simulink model "SystemSimulationPPO"  (R2024b)
settings: Solver=FixedStepAuto  StartTime=0.0  StopTime=TMax  FixedStep=0.01  MaxStep=DT  RelTol=1e-3  EnableMultiTasking=on
undefined symbols (not defined in the file or in its folder): Beta_Array, Cp_Table, Ct_Table, MPC_Implicit, MPC_Lidar, OutList, strmatch, TSR_Array
libraries: simulink_extras x3, rllib x1, matrix_library x1
settings Model: Creator=bjonkman  LastModifiedBy=malth
settings SolverCC: AlgebraicLoopSolver=TrustRegion  AutoInsertRateTranBlk=on
settings DataIOCC: SaveFormat=Array  SignalLoggingSaveFormat=ModelDataLogs  SaveOutput=off  SaveTime=off  ReturnWorkspaceOutputs=off  SignalLoggingName=sigsOut
settings OptimizationCC: ExpressionDepthLimit=2147483647  LifeSpan=inf
settings DebuggingCC: SaveWithParameterizedLinksMsg=none  UnderspecifiedInitializationDetection=Classic  MergeDetectMultiDrivingBlocksExec=none  SignalResolutionControl=TryResolveAllWithWarning  MultiTaskDSMMsg=warning  MultiTaskCondExecSysMsg=none  FcnCallInpInsideContextMsg=warning  UnconnectedInputMsg=warning  UnconnectedOutputMsg=warning  UnconnectedLineMsg=warning  StateNameClashWarn=warning  SFUnexpectedBacktrackingDiag=warning  SFNoUnconditionalDefaultTransitionDiag=warning  SFExecutionAtInitializationDiag=none  UnderSpecifiedDimensionMsg=warning  ArithmeticOperatorsInVariantConditions=warning
settings HardwareCC: ProdBitPerPointer=32  ProdBitPerSizeT=32  ProdBitPerPtrDiffT=32  ProdLargestAtomicFloat=None  ProdIntDivRoundTo=Undefined  ProdEndianess=Unspecified  ProdWordSize=32  ProdHWDeviceType=32-bit Generic  TargetBitPerPointer=64  TargetBitPerSizeT=64  TargetBitPerPtrDiffT=64  TargetLongLongMode=on  TargetIntDivRoundTo=Zero  TargetEndianess=LittleEndian  TargetWordSize=64  TargetHWDeviceType=MATLAB Host  ProdEqTarget=off
settings ModelReferenceCC: EnableRefExpFcnMdlSchedulingChecks=on  PropagateSignalLabelsOutOfModel=off
settings SFSimCC: SimUseLocalCustomCode=off  CustomCodeUndefinedFunction=UseInterfaceOnly
settings RTWCC: RTWUseLocalCustomCode=off  GPUComputeCapability=3.5  DLArmComputeVersion=19.05
settings CodeAppCC: StateflowObjectComments=on
settings GRTTargetCC: TargetLangStandard=C89/C90 (ANSI)  ModelReferenceCompliant=off  ParMdlRefBuildCompliant=off  CompOptLevelCompliant=off  ConcurrentExecutionCompliant=off  CombineOutputUpdateFcns=off  MatFileLogging=off  GRTInterface=on
settings ConfigComp: CovMetricSettings=dw  CovSaveCumulativeToWorkspaceVar=on  CovSaveSingleToWorkspaceVar=on  CovExternalEMLEnable=off

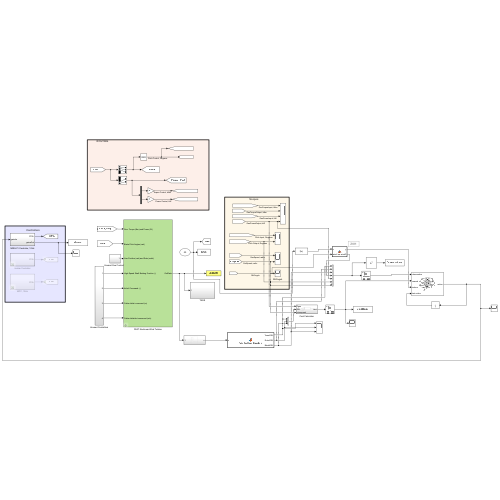
[thumbnail: Simulink's stored preview of the top-level diagram]
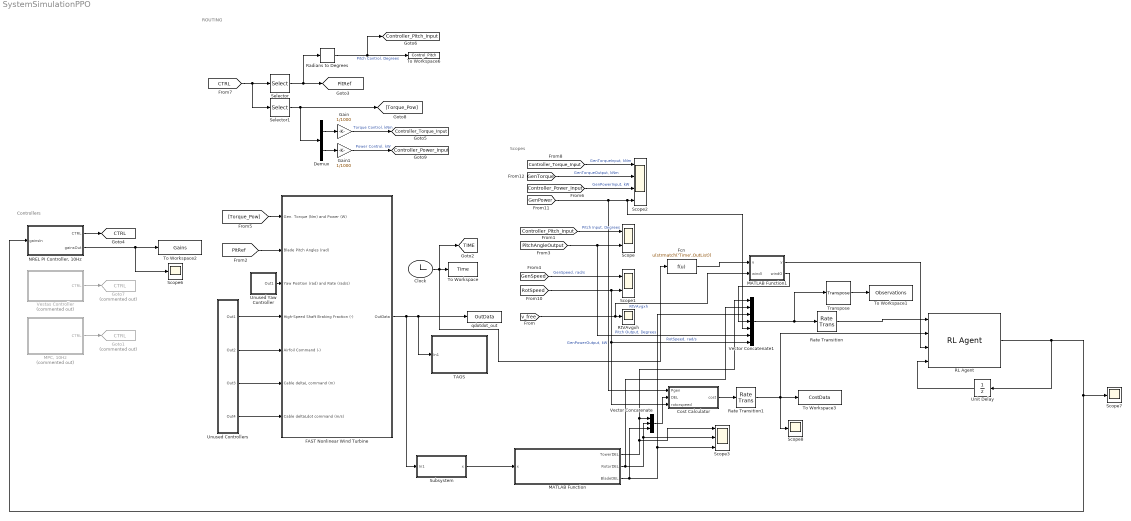
== system SystemSimulationPPO ==
  note: ROUTING
  note: Scopes
  note: Controllers
  Clock : Clock
  Cost Calculator : Subsystem
  Demux : Demux  Outputs=2
  FAST Nonlinear Wind Turbine : Subsystem  mask(FAST Nonlinear Wind Turbine){}
      mask help: This block contains the FAST S-Function.
      mask init:
      | clear FAST_SFunc
  Fcn : Fcn  Expr=u(strmatch('Time',OutList))
  Gain : Gain  Gain=1/1000
  Gain1 : Gain  Gain=1/1000
  Goto1 : Goto  Commented=on  GotoTag=CTRL  TagVisibility=global
  Goto7 : Goto  Commented=on  GotoTag=CTRL  TagVisibility=global
  MATLAB Function : MATLAB Function  TreatAsAtomicUnit=on
  MATLAB Function1 : MATLAB Function  TreatAsAtomicUnit=on
  "MPC, 10Hz" : Subsystem  Commented=on
  "NREL PI Controller, 10Hz" : Subsystem
  RL Agent : rllib/RL Agent  Agent=agent  ExternalActionAsInput=off  ProvideLastAction=on  ProvideCumRwd=off  TreatAsDirectFeedthrough=on  UseStrictObservationDataTypes=off
  Radians to Degrees : simulink_extras/Transformations/Radians to Degrees
  Rate Transition : RateTransition  OutPortSampleTime=0.1
  Rate Transition1 : RateTransition  OutPortSampleTime=0.1
  RtVAvgxh : Scope
  Scope : Scope  NumInputPorts=2
  Scope1 : Scope  NumInputPorts=2
  Scope2 : Scope  NumInputPorts=4
  Scope3 : Scope  NumInputPorts=3
  Scope6 : Scope
  Scope7 : Scope
  Scope8 : Scope
  Selector : Selector  InputPortWidth=5  IndexOptions=Index vector (dialog)  Indices=[1, 2, 3]  OutputSizes=1
  Selector1 : Selector  InputPortWidth=5  IndexOptions=Index vector (dialog)  Indices=[4, 5]  OutputSizes=1
  Subsystem : Subsystem
  TAGS : Subsystem
  To Workspace : ToWorkspace  VariableName=Time  SampleTime=-1
  To Workspace1 : ToWorkspace  VariableName=Observations  SampleTime=-1
      settings: Save2DSignal=2-D array (concatenate along first dimension)
  To Workspace2 : ToWorkspace  VariableName=Gains  SaveFormat=Timeseries  SampleTime=-1
  To Workspace3 : ToWorkspace  VariableName=CostData  SampleTime=-1
  To Workspace6 : ToWorkspace  VariableName=Control_Pitch  SampleTime=-1
  Transpose : matrix_library/Transpose
  Unit Delay : UnitDelay  SampleTime=-1  HasFrameUpgradeWarning=on
  Unused Controllers : Subsystem
  Unused Yaw Controller : Subsystem
  Vector Concatenate : Concatenate  NumInputs=3  Mode=Multidimensional array  ConcatenateDimension=2
  Vector Concatenate1 : Concatenate  NumInputs=7  Mode=Multidimensional array  ConcatenateDimension=2
  Vestas Controller : Subsystem  Commented=on  TreatAsAtomicUnit=on  SystemSampleTime=0.01
  qdotdot_out : ToWorkspace  VariableName=OutData  SampleTime=-1
  tag scope: CTRL=global, Controller_Pitch_Input=global, Controller_Power_Input=global, Controller_Torque_Input=global, PitRef=global, TIME=global
  wires:
  Clock/1 -> [TIME], To Workspace/1, Fcn/1
  Unused Yaw Controller/1(Out1) -> FAST Nonlinear Wind Turbine/3(Yaw Position (rad) and Rate (rad/s))
  [PitRef] -> FAST Nonlinear Wind Turbine/2(Blade Pitch Angles (rad))
  [PitchAngleOutput] -> Vector Concatenate1/6, Scope/2  "Pitch Output, Degrees"
  [GenSpeed] -> Scope1/1  "GenSpeed, rad/s"
  [RotSpeed] -> Cost Calculator/3(rotorspeed), Vector Concatenate1/7, Scope1/2  "RotSpeed, rad/s"
  [v_free] -> RtVAvgxh/1, MATLAB Function1/2(windI)  "RtVAvgxh"
  "NREL PI Controller, 10Hz"/1(CTRL) -> [CTRL]
  [Controller_Pitch_Input] -> Scope/1  "Pitch Input, Degrees"
  Unused Controllers/1(Out1) -> FAST Nonlinear Wind Turbine/4(High-Speed Shaft Braking Fraction (-))
  Unused Controllers/2(Out2) -> FAST Nonlinear Wind Turbine/5(Airfoil Command (-))
  Unused Controllers/3(Out3) -> FAST Nonlinear Wind Turbine/6(Cable deltaL command (m))
  Unused Controllers/4(Out4) -> FAST Nonlinear Wind Turbine/7(Cable deltaLdot command (m/s))
  "MPC, 10Hz"/1(CTRL) -> Goto1/1
  Vestas Controller/1(CTRL) -> Goto7/1
  [Torque_Pow] -> FAST Nonlinear Wind Turbine/1(Gen. Torque (Nm) and Power (W))
  [CTRL] -> Selector1/1, Selector/1
  Selector/1 -> Radians to Degrees/1, [PitRef]
  Radians to Degrees/1 -> [Controller_Pitch_Input], To Workspace6/1  "Pitch Control, Degrees"
  Selector1/1 -> Demux/1, [Torque_Pow]
  [GenTorque] -> Scope2/2  "GenTorqueOutput, kNm"
  [GenPower] -> Cost Calculator/1(Pgen), Vector Concatenate1/5, Scope2/4  "GenPowerOutput, kW"
  Demux/1 -> Gain/1
  [Controller_Power_Input] -> Scope2/3  "GenPowerInput, kW"
  [Controller_Torque_Input] -> Scope2/1  "GenTorqueInput, kNm"
  Gain/1 -> [Controller_Torque_Input]  "Torque Control, kNm"
  Gain1/1 -> [Controller_Power_Input]  "Power Control, kW"
  Demux/2 -> Gain1/1
  Subsystem/1(x) -> MATLAB Function/1(x)
  Vector Concatenate/1 -> Cost Calculator/2(DEL)
  MATLAB Function/1(TowerDEL) -> Scope3/1, Vector Concatenate1/1, Vector Concatenate/1
  MATLAB Function/2(RotorDEL) -> Vector Concatenate1/2, Scope3/2, Vector Concatenate/2
  MATLAB Function/3(BladeDEL) -> Vector Concatenate/3, Scope3/3, Vector Concatenate1/3
  "NREL PI Controller, 10Hz"/2(gainsOut) -> Scope6/1, To Workspace2/1
  RL Agent/1 -> Unit Delay/1, "NREL PI Controller, 10Hz"/1(gainsIn), Scope7/1
  Transpose/1 -> To Workspace1/1
  FAST Nonlinear Wind Turbine/1(OutData) -> qdotdot_out/1, TAGS/1(In1), Subsystem/1(In1)
  Vector Concatenate1/1 -> Rate Transition/1, Transpose/1
  Cost Calculator/1(cost) -> Rate Transition1/1
  Rate Transition/1 -> RL Agent/1
  Rate Transition1/1 -> RL Agent/2, To Workspace3/1, Scope8/1
  MATLAB Function1/1(y) -> RL Agent/3
  Fcn/1 -> MATLAB Function1/1(u)
  MATLAB Function1/2(windO) -> Vector Concatenate1/4
  Unit Delay/1 -> RL Agent/4

== system SystemSimulationPPO/Cost Calculator ==
  Pgen : Inport
  DEL : Inport  Port=2
  rotorspeed : Inport  Port=3
  MATLAB Function : MATLAB Function  TreatAsAtomicUnit=on
  cost : Outport
  wires:
  Pgen/1 -> MATLAB Function/2(Pgen)
  DEL/1 -> MATLAB Function/1(DEL)
  MATLAB Function/1(cost) -> cost/1
  rotorspeed/1 -> MATLAB Function/3(rotorspeed)

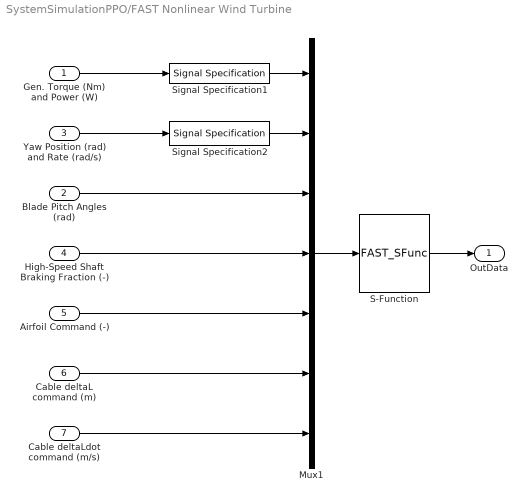
== system SystemSimulationPPO/FAST Nonlinear Wind Turbine ==
  Gen. Torque (Nm) and Power (W) : Inport
  Blade Pitch Angles (rad) : Inport  Port=2
  Yaw Position (rad) and Rate (rad/s) : Inport  Port=3
  High-Speed Shaft Braking Fraction (-) : Inport  Port=4
  Airfoil Command (-) : Inport  Port=5
  Cable deltaL command (m) : Inport  Port=6
  Cable deltaLdot command (m/s) : Inport  Port=7
  Mux1 : Mux  Inputs=7
  S-Function : S-Function  FunctionName=FAST_SFunc  Parameters=FAST_InputFileName, TMax, 0  SFunctionDeploymentMode=off  EnableBusSupport=off
  Signal Specification1 : SignalSpecification  OutDataTypeStr=double  Dimensions=2
  Signal Specification2 : SignalSpecification  OutDataTypeStr=double  Dimensions=2
  OutData : Outport
  wires:
  Gen. Torque (Nm) and Power (W)/1 -> Signal Specification1/1
  S-Function/1 -> OutData/1
  Mux1/1 -> S-Function/1
  Blade Pitch Angles (rad)/1 -> Mux1/3
  Yaw Position (rad) and Rate (rad/s)/1 -> Signal Specification2/1
  Signal Specification1/1 -> Mux1/1
  Signal Specification2/1 -> Mux1/2
  High-Speed Shaft Braking Fraction (-)/1 -> Mux1/4
  Airfoil Command (-)/1 -> Mux1/5
  Cable deltaL command (m)/1 -> Mux1/6
  Cable deltaLdot command (m/s)/1 -> Mux1/7

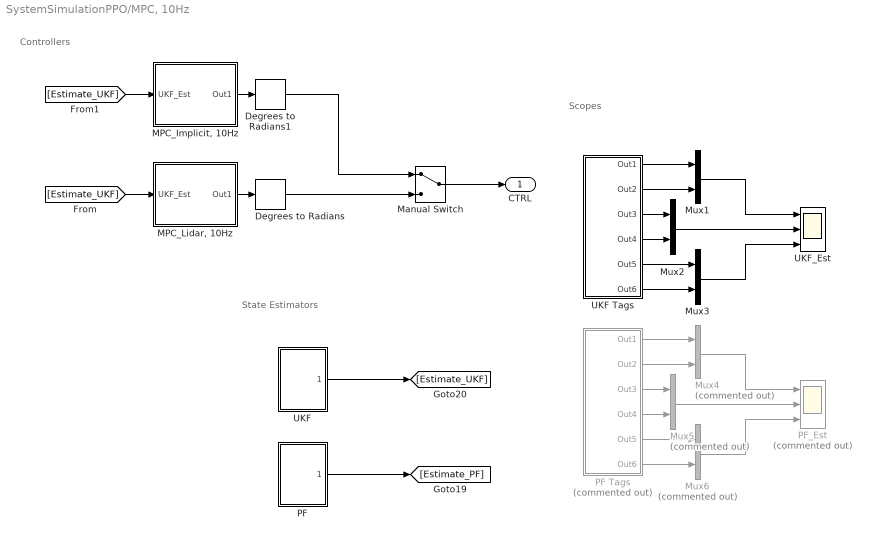
== system SystemSimulationPPO/MPC, 10Hz ==
  note: State Estimators
  note: Scopes
  note: Controllers
  Degrees to Radians : simulink_extras/Transformations/Degrees to Radians
  Degrees to Radians1 : simulink_extras/Transformations/Degrees to Radians
  "MPC_Implicit, 10Hz" : Subsystem
  "MPC_Lidar, 10Hz" : Subsystem
  Manual Switch : ManualSwitch
  Mux1 : Mux  Inputs=2
  Mux2 : Mux  Inputs=2
  Mux3 : Mux  Inputs=2
  Mux4 : Mux  Commented=on  Inputs=2
  Mux5 : Mux  Commented=on  Inputs=2
  Mux6 : Mux  Commented=on  Inputs=2
  PF : Subsystem
  PF Tags : Subsystem  Commented=on
  PF_Est : Scope  Commented=on  NumInputPorts=3
  UKF : Subsystem
  UKF Tags : Subsystem
  UKF_Est : Scope  NumInputPorts=3
  CTRL : Outport
  wires:
  UKF/1(estimate) -> [Estimate_UKF]
  PF/1(estimate) -> [Estimate_PF]
  "MPC_Implicit, 10Hz"/1(Out1) -> Degrees to Radians1/1
  Degrees to Radians1/1 -> Manual Switch/1
  "MPC_Lidar, 10Hz"/1(Out1) -> Degrees to Radians/1
  Degrees to Radians/1 -> Manual Switch/2
  Manual Switch/1 -> CTRL/1
  [Estimate_UKF] -> "MPC_Lidar, 10Hz"/1(UKF_Est)
  [Estimate_UKF] -> "MPC_Implicit, 10Hz"/1(UKF_Est)
  Mux2/1 -> UKF_Est/2
  Mux4/1 -> PF_Est/1
  PF Tags/3(Out3) -> Mux5/1
  Mux6/1 -> PF_Est/3
  PF Tags/1(Out1) -> Mux4/1
  PF Tags/4(Out4) -> Mux5/2
  Mux5/1 -> PF_Est/2
  UKF Tags/2(Out2) -> Mux1/2
  PF Tags/5(Out5) -> Mux6/1
  Mux3/1 -> UKF_Est/3
  UKF Tags/5(Out5) -> Mux3/1
  UKF Tags/4(Out4) -> Mux2/2
  UKF Tags/1(Out1) -> Mux1/1
  Mux1/1 -> UKF_Est/1
  PF Tags/2(Out2) -> Mux4/2
  UKF Tags/3(Out3) -> Mux2/1
  UKF Tags/6(Out6) -> Mux3/2
  PF Tags/6(Out6) -> Mux6/2

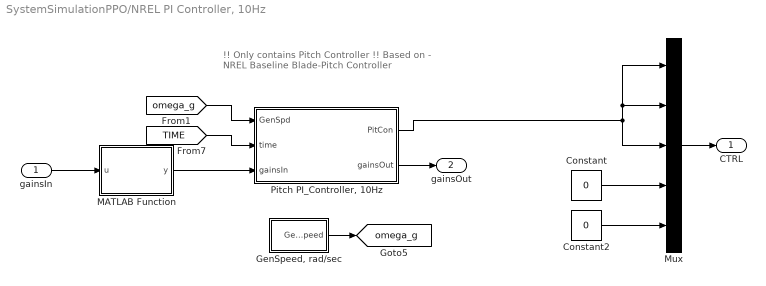
== system SystemSimulationPPO/NREL PI Controller, 10Hz ==
  note: !! Only contains Pitch Controller !!
      |
      | Based on
      | - NREL Baseline Blade-Pitch Controller
  gainsIn : Inport
  Constant : Constant  Value=0
  Constant2 : Constant  Value=0
  "GenSpeed, rad/sec" : Subsystem
  MATLAB Function : MATLAB Function  TreatAsAtomicUnit=on
  Mux : Mux  Inputs=5
  "Pitch PI_Controller, 10Hz" : MATLAB Function  TreatAsAtomicUnit=on
  CTRL : Outport
  gainsOut : Outport  Port=2
  tag scope: omega_g=global
  wires:
  [omega_g] -> "Pitch PI_Controller, 10Hz"/1(GenSpd)
  [TIME] -> "Pitch PI_Controller, 10Hz"/2(time)
  "Pitch PI_Controller, 10Hz"/1(PitCon) -> Mux/3, Mux/2, Mux/1
  Mux/1 -> CTRL/1
  "GenSpeed, rad/sec"/1(GenSpeed) -> [omega_g]
  Constant/1 -> Mux/4
  Constant2/1 -> Mux/5
  gainsIn/1 -> MATLAB Function/1(u)
  "Pitch PI_Controller, 10Hz"/2(gainsOut) -> gainsOut/1
  MATLAB Function/1(y) -> "Pitch PI_Controller, 10Hz"/3(gainsIn)

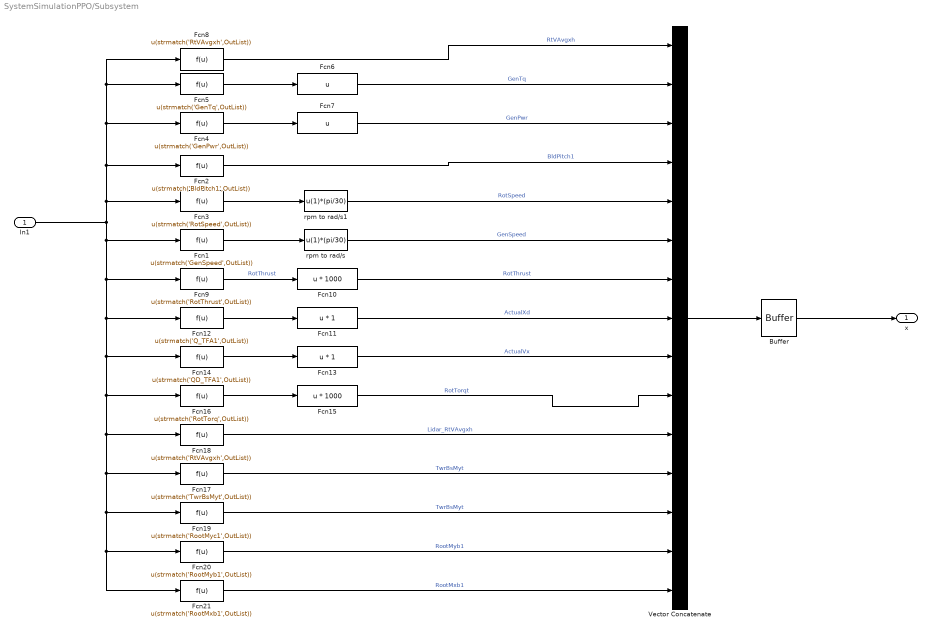
== system SystemSimulationPPO/Subsystem ==
  In1 : Inport
  Buffer : Buffer  N=10  V=9  OutputFrames=off
  Fcn1 : Fcn  Expr=u(strmatch('GenSpeed',OutList))
  Fcn10 : Fcn  Expr=u * 1000
  Fcn11 : Fcn  Expr=u * 1
  Fcn12 : Fcn  Expr=u(strmatch('Q_TFA1',OutList))
  Fcn13 : Fcn  Expr=u * 1
  Fcn14 : Fcn  Expr=u(strmatch('QD_TFA1',OutList))
  Fcn15 : Fcn  Expr=u * 1000
  Fcn16 : Fcn  Expr=u(strmatch('RotTorq',OutList))
  Fcn17 : Fcn  Expr=u(strmatch('TwrBsMyt',OutList))
  Fcn18 : Fcn  Expr=u(strmatch('RtVAvgxh',OutList))
  Fcn19 : Fcn  Expr=u(strmatch('RootMyc1',OutList))
  Fcn2 : Fcn  Expr=u(strmatch('BldPitch1',OutList))
  Fcn20 : Fcn  Expr=u(strmatch('RootMyb1',OutList))
  Fcn21 : Fcn  Expr=u(strmatch('RootMxb1',OutList))
  Fcn3 : Fcn  Expr=u(strmatch('RotSpeed',OutList))
  Fcn4 : Fcn  Expr=u(strmatch('GenPwr',OutList))
  Fcn5 : Fcn  Expr=u(strmatch('GenTq',OutList))
  Fcn6 : Fcn  Expr=u
  Fcn7 : Fcn  Expr=u
  Fcn8 : Fcn  Expr=u(strmatch('RtVAvgxh',OutList))
  Fcn9 : Fcn  Expr=u(strmatch('RotThrust',OutList))
  Vector Concatenate : Concatenate  NumInputs=15  Mode=Multidimensional array  ConcatenateDimension=2
  rpm to rad/s : Fcn  Expr=u(1)*(pi/30)
  rpm to rad/s1 : Fcn  Expr=u(1)*(pi/30)
  x : Outport
  wires:
  Fcn16/1 -> Fcn15/1
  Fcn8/1 -> Vector Concatenate/1  "RtVAvgxh"
  Fcn6/1 -> Vector Concatenate/2  "GenTq"
  Fcn4/1 -> Fcn7/1
  In1/1 -> Fcn8/1, Fcn5/1, Fcn4/1, Fcn2/1, Fcn3/1, Fcn21/1, Fcn20/1, Fcn19/1, Fcn17/1, Fcn18/1, Fcn16/1, Fcn14/1, Fcn12/1, Fcn9/1, Fcn1/1
  Fcn14/1 -> Fcn13/1
  Fcn17/1 -> Vector Concatenate/12  "TwrBsMyt"
  rpm to rad/s/1 -> Vector Concatenate/6  "GenSpeed"
  Fcn5/1 -> Fcn6/1
  Fcn13/1 -> Vector Concatenate/9  "ActualVx"
  Fcn1/1 -> rpm to rad/s/1
  Fcn18/1 -> Vector Concatenate/11  "Lidar_RtVAvgxh"
  Fcn19/1 -> Vector Concatenate/13  "TwrBsMyt"
  Fcn10/1 -> Vector Concatenate/7  "RotThrust"
  rpm to rad/s1/1 -> Vector Concatenate/5  "RotSpeed"
  Fcn20/1 -> Vector Concatenate/14  "RootMyb1"
  Fcn12/1 -> Fcn11/1
  Fcn11/1 -> Vector Concatenate/8  "ActualXd"
  Fcn15/1 -> Vector Concatenate/10  "RotTorqt"
  Fcn9/1 -> Fcn10/1  "RotThrust"
  Fcn7/1 -> Vector Concatenate/3  "GenPwr"
  Fcn2/1 -> Vector Concatenate/4  "BldPitch1"
  Fcn21/1 -> Vector Concatenate/15  "RootMxb1"
  Fcn3/1 -> rpm to rad/s1/1
  Vector Concatenate/1 -> Buffer/1
  Buffer/1 -> x/1

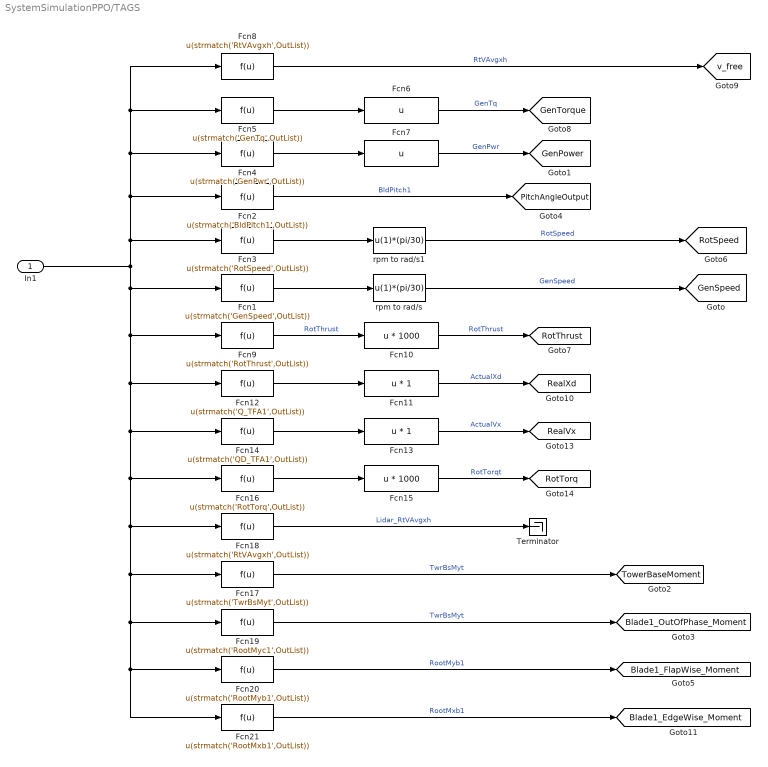
== system SystemSimulationPPO/TAGS ==
  In1 : Inport
  Fcn1 : Fcn  Expr=u(strmatch('GenSpeed',OutList))
  Fcn10 : Fcn  Expr=u * 1000
  Fcn11 : Fcn  Expr=u * 1
  Fcn12 : Fcn  Expr=u(strmatch('Q_TFA1',OutList))
  Fcn13 : Fcn  Expr=u * 1
  Fcn14 : Fcn  Expr=u(strmatch('QD_TFA1',OutList))
  Fcn15 : Fcn  Expr=u * 1000
  Fcn16 : Fcn  Expr=u(strmatch('RotTorq',OutList))
  Fcn17 : Fcn  Expr=u(strmatch('TwrBsMyt',OutList))
  Fcn18 : Fcn  Expr=u(strmatch('RtVAvgxh',OutList))
  Fcn19 : Fcn  Expr=u(strmatch('RootMyc1',OutList))
  Fcn2 : Fcn  Expr=u(strmatch('BldPitch1',OutList))
  Fcn20 : Fcn  Expr=u(strmatch('RootMyb1',OutList))
  Fcn21 : Fcn  Expr=u(strmatch('RootMxb1',OutList))
  Fcn3 : Fcn  Expr=u(strmatch('RotSpeed',OutList))
  Fcn4 : Fcn  Expr=u(strmatch('GenPwr',OutList))
  Fcn5 : Fcn  Expr=u(strmatch('GenTq',OutList))
  Fcn6 : Fcn  Expr=u
  Fcn7 : Fcn  Expr=u
  Fcn8 : Fcn  Expr=u(strmatch('RtVAvgxh',OutList))
  Fcn9 : Fcn  Expr=u(strmatch('RotThrust',OutList))
  Terminator : Terminator
  rpm to rad/s : Fcn  Expr=u(1)*(pi/30)
  rpm to rad/s1 : Fcn  Expr=u(1)*(pi/30)
  tag scope: Blade1_EdgeWise_Moment=global, Blade1_FlapWise_Moment=global, Blade1_OutOfPhase_Moment=global, GenPower=global, GenSpeed=global, GenTorque=global, PitchAngleOutput=global, RealVx=global, RealXd=global, RotSpeed=global, RotThrust=global, RotTorq=global, TowerBaseMoment=global, v_free=global
  wires:
  rpm to rad/s/1 -> [GenSpeed]  "GenSpeed"
  Fcn1/1 -> rpm to rad/s/1
  Fcn3/1 -> rpm to rad/s1/1
  Fcn11/1 -> [RealXd]  "ActualXd"
  In1/1 -> Fcn8/1, Fcn5/1, Fcn4/1, Fcn2/1, Fcn3/1, Fcn21/1, Fcn20/1, Fcn19/1, Fcn17/1, Fcn18/1, Fcn16/1, Fcn14/1, Fcn12/1, Fcn9/1, Fcn1/1
  Fcn7/1 -> [GenPower]  "GenPwr"
  Fcn16/1 -> Fcn15/1
  Fcn10/1 -> [RotThrust]  "RotThrust"
  Fcn6/1 -> [GenTorque]  "GenTq"
  rpm to rad/s1/1 -> [RotSpeed]  "RotSpeed"
  Fcn8/1 -> [v_free]  "RtVAvgxh"
  Fcn5/1 -> Fcn6/1
  Fcn13/1 -> [RealVx]  "ActualVx"
  Fcn4/1 -> Fcn7/1
  Fcn14/1 -> Fcn13/1
  Fcn15/1 -> [RotTorq]  "RotTorqt"
  Fcn2/1 -> [PitchAngleOutput]  "BldPitch1"
  Fcn9/1 -> Fcn10/1  "RotThrust"
  Fcn12/1 -> Fcn11/1
  Fcn18/1 -> Terminator/1  "Lidar_RtVAvgxh"
  Fcn17/1 -> [TowerBaseMoment]  "TwrBsMyt"
  Fcn20/1 -> [Blade1_FlapWise_Moment]  "RootMyb1"
  Fcn21/1 -> [Blade1_EdgeWise_Moment]  "RootMxb1"
  Fcn19/1 -> [Blade1_OutOfPhase_Moment]  "TwrBsMyt"

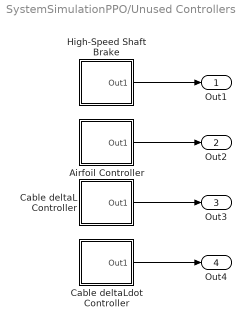
== system SystemSimulationPPO/Unused Controllers ==
  Airfoil Controller : Subsystem
  Cable deltaL Controller : Subsystem
  Cable deltaLdot Controller : Subsystem
  High-Speed Shaft Brake : Subsystem
  Out1 : Outport
  Out2 : Outport  Port=2
  Out3 : Outport  Port=3
  Out4 : Outport  Port=4
  wires:
  Airfoil Controller/1(Out1) -> Out2/1
  High-Speed Shaft Brake/1(Out1) -> Out1/1
  Cable deltaLdot Controller/1(Out1) -> Out4/1
  Cable deltaL Controller/1(Out1) -> Out3/1

== system SystemSimulationPPO/Unused Yaw Controller ==
  Mux : Mux  Inputs=2
  Yaw Position : Constant  Value=0
  Yaw rate : Constant  Value=0
  Out1 : Outport
  wires:
  Mux/1 -> Out1/1
  Yaw Position/1 -> Mux/1
  Yaw rate/1 -> Mux/2

== system SystemSimulationPPO/Vestas Controller ==
  CTRL : Outport

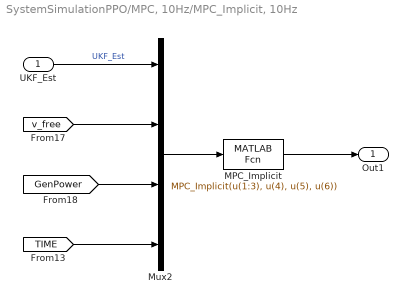
== system SystemSimulationPPO/MPC, 10Hz/MPC_Implicit, 10Hz ==
  UKF_Est : Inport
  MPC_Implicit : MATLABFcn  MATLABFcn=MPC_Implicit(u(1:3), u(4), u(5), u(6))
  Mux2 : Mux
  Out1 : Outport
  wires:
  Mux2/1 -> MPC_Implicit/1
  [GenPower] -> Mux2/3
  [v_free] -> Mux2/2
  [TIME] -> Mux2/4
  MPC_Implicit/1 -> Out1/1
  UKF_Est/1 -> Mux2/1  "UKF_Est"

== system SystemSimulationPPO/MPC, 10Hz/MPC_Lidar, 10Hz ==
  UKF_Est : Inport
  MPC_Lidar : MATLABFcn  MATLABFcn=MPC_Lidar(u(1:3), u(4), u(5), u(6))
  Mux2 : Mux
  Out1 : Outport
  wires:
  Mux2/1 -> MPC_Lidar/1
  [GenPower] -> Mux2/3
  [v_free] -> Mux2/2
  [TIME] -> Mux2/4
  MPC_Lidar/1 -> Out1/1
  UKF_Est/1 -> Mux2/1  "UKF_Est"

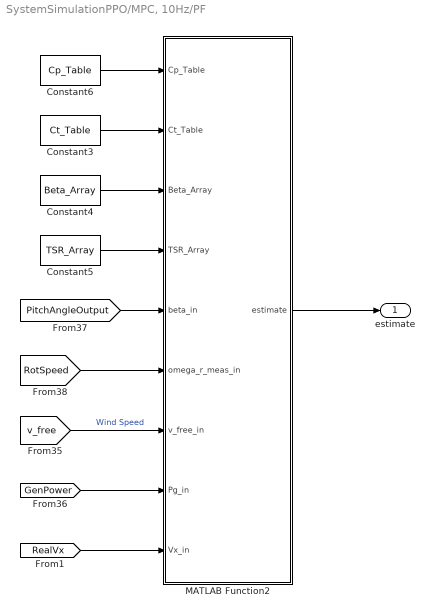
== system SystemSimulationPPO/MPC, 10Hz/PF ==
  Constant3 : Constant  Value=Ct_Table  SampleTime=-1
  Constant4 : Constant  Value=Beta_Array  SampleTime=-1
  Constant5 : Constant  Value=TSR_Array  SampleTime=-1
  Constant6 : Constant  Value=Cp_Table  SampleTime=-1
  MATLAB Function2 : MATLAB Function  TreatAsAtomicUnit=on
  estimate : Outport
  wires:
  [v_free] -> MATLAB Function2/7(v_free_in)  "Wind Speed"
  Constant6/1 -> MATLAB Function2/1(Cp_Table)
  Constant3/1 -> MATLAB Function2/2(Ct_Table)
  Constant4/1 -> MATLAB Function2/3(Beta_Array)
  [GenPower] -> MATLAB Function2/8(Pg_in)
  Constant5/1 -> MATLAB Function2/4(TSR_Array)
  [PitchAngleOutput] -> MATLAB Function2/5(beta_in)
  [RotSpeed] -> MATLAB Function2/6(omega_r_meas_in)
  MATLAB Function2/1(estimate) -> estimate/1
  [RealVx] -> MATLAB Function2/9(Vx_in)

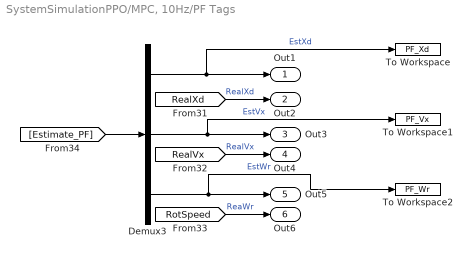
== system SystemSimulationPPO/MPC, 10Hz/PF Tags ==
  Demux3 : Demux  Outputs=3
  To Workspace : ToWorkspace  VariableName=PF_Xd  SampleTime=-1
  To Workspace1 : ToWorkspace  VariableName=PF_Vx  SampleTime=-1
  To Workspace2 : ToWorkspace  VariableName=PF_Wr  SampleTime=-1
  Out1 : Outport
  Out2 : Outport  Port=2
  Out3 : Outport  Port=3
  Out4 : Outport  Port=4
  Out5 : Outport  Port=5
  Out6 : Outport  Port=6
  wires:
  Demux3/1 -> Out1/1, To Workspace/1  "EstXd"
  [RotSpeed] -> Out6/1  "ReaWr"
  [RealVx] -> Out4/1  "RealVx"
  [RealXd] -> Out2/1  "RealXd"
  Demux3/3 -> Out5/1, To Workspace2/1  "EstWr"
  Demux3/2 -> Out3/1, To Workspace1/1  "EstVx"
  [Estimate_PF] -> Demux3/1

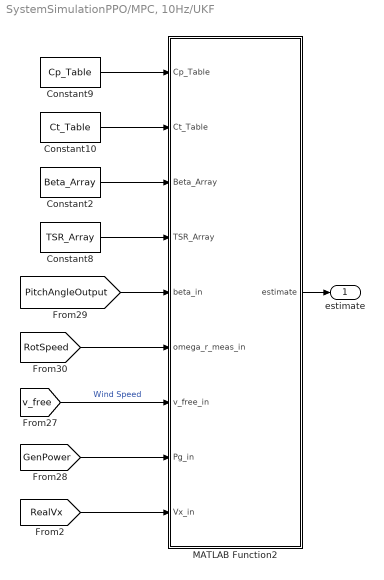
== system SystemSimulationPPO/MPC, 10Hz/UKF ==
  Constant10 : Constant  Value=Ct_Table  SampleTime=-1
  Constant2 : Constant  Value=Beta_Array  SampleTime=-1
  Constant8 : Constant  Value=TSR_Array  SampleTime=-1
  Constant9 : Constant  Value=Cp_Table  SampleTime=-1
  MATLAB Function2 : MATLAB Function  TreatAsAtomicUnit=on
  estimate : Outport
  wires:
  [GenPower] -> MATLAB Function2/8(Pg_in)
  [RotSpeed] -> MATLAB Function2/6(omega_r_meas_in)
  Constant8/1 -> MATLAB Function2/4(TSR_Array)
  [v_free] -> MATLAB Function2/7(v_free_in)  "Wind Speed"
  Constant2/1 -> MATLAB Function2/3(Beta_Array)
  Constant9/1 -> MATLAB Function2/1(Cp_Table)
  Constant10/1 -> MATLAB Function2/2(Ct_Table)
  [PitchAngleOutput] -> MATLAB Function2/5(beta_in)
  MATLAB Function2/1(estimate) -> estimate/1
  [RealVx] -> MATLAB Function2/9(Vx_in)

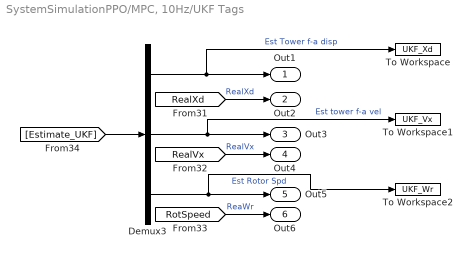
== system SystemSimulationPPO/MPC, 10Hz/UKF Tags ==
  Demux3 : Demux  Outputs=3
  To Workspace : ToWorkspace  VariableName=UKF_Xd  SampleTime=-1
  To Workspace1 : ToWorkspace  VariableName=UKF_Vx  SampleTime=-1
  To Workspace2 : ToWorkspace  VariableName=UKF_Wr  SampleTime=-1
  Out1 : Outport
  Out2 : Outport  Port=2
  Out3 : Outport  Port=3
  Out4 : Outport  Port=4
  Out5 : Outport  Port=5
  Out6 : Outport  Port=6
  wires:
  Demux3/1 -> Out1/1, To Workspace/1  "Est Tower f-a disp"
  [RotSpeed] -> Out6/1  "ReaWr"
  [RealVx] -> Out4/1  "RealVx"
  [RealXd] -> Out2/1  "RealXd"
  Demux3/3 -> Out5/1, To Workspace2/1  "Est Rotor Spd"
  Demux3/2 -> Out3/1, To Workspace1/1  "Est tower f-a vel"
  [Estimate_UKF] -> Demux3/1

== system SystemSimulationPPO/NREL PI Controller, 10Hz/GenSpeed, rad//sec ==
  MATLAB Function5 : MATLAB Function  TreatAsAtomicUnit=on
  GenSpeed : Outport
  wires:
  [RotSpeed] -> MATLAB Function5/1(omega_r)  "ReaWr"
  MATLAB Function5/1(GenSpeed) -> GenSpeed/1

== system SystemSimulationPPO/Unused Controllers/Airfoil Controller ==
  Airfoil command : Constant  Value=zeros(1,3)'
  Out1 : Outport
  wires:
  Airfoil command/1 -> Out1/1

== system SystemSimulationPPO/Unused Controllers/Cable deltaL Controller ==
  Cable deltaL command : Constant  Value=zeros(1,20)'
  Out1 : Outport
  wires:
  Cable deltaL command/1 -> Out1/1

== system SystemSimulationPPO/Unused Controllers/Cable deltaLdot Controller ==
  Cable deltaLdot command : Constant  Value=zeros(1,20)'
  Out1 : Outport
  wires:
  Cable deltaLdot command/1 -> Out1/1

== system SystemSimulationPPO/Unused Controllers/High-Speed Shaft Brake ==
  High-Speed Shaft Braking Fraction : Constant  Value=0
  Out1 : Outport
  wires:
  High-Speed Shaft Braking Fraction/1 -> Out1/1

== matlab function SystemSimulationPPO/NREL PI Controller, 10Hz/Pitch PI_Controller, 10Hz ==
  data: GenSpd input; PitCon output; time input; gainsIn input; gainsOut output
function [PitCon,gainsOut]  = PI(GenSpd, time, gainsIn)%, delta_Kp, delta_Ki) %,OUTKp,OUTKi

persistent n dt j;
persistent MaxPit MinPit MaxPitRat beta_K IntSpdErr Kp Ki;
persistent RefGenSpd beta;

if isempty(n)
    n = 1;

    dt = 0.1;                                                               % Controller sampling frequency = 1/dt
    
    beta_K = 6.302336 * pi/180;                                              % the blade-pitch angle at which the pitch sensitivity has doubled from its value at the rated operating point (beta = 0)
     
    MaxPit = 45 * pi/180;                                                       % Maximum pitch, rad
    MinPit = 0 * pi/180;                                                        % Minimum pitch, rad
    MaxPitRat = 8 * pi/180;                                                     % Pitch rate, rad/s

    RatedRotorSpeed = 12.1 * pi/30;
    RatedPower = 5296610.0;
    J_Drivetrain = 4.3786e+07;
    zeta_PI = 0.67;                                                          % Damping ratio of PI controller modeled as 2nd order system, recommended 0.6-0.7
    wn = 0.83;                                                               % Natural Angular frequency, recommended 0.6, rad/s, wn = 2*pi* eigen frequency
    N = 97;                                                                 % Gear Ratio, drivetrain
    partPower_partBeta = -25.52e6;                                          % pitch sensitivity at rated operating point (beta = 0), watt/rad
    Kp = ( 2 * J_Drivetrain * RatedRotorSpeed * zeta_PI * wn - RatedPower/RatedRotorSpeed ) / ( N * (-1) * partPower_partBeta );
    Ki = ( J_Drivetrain * RatedRotorSpeed * wn^2 ) / ( N * (-1) * partPower_partBeta );
    gainsOut = [Kp; Ki];
    RefGenSpd = RatedRotorSpeed * 97;
    beta = 12 * pi/180;
    IntSpdErr = 0;
end

t = time;

if mod(t, dt)== 0
    gainsOut = gainsIn;
    Kp = gainsOut(1);
    Ki = gainsOut(2);
    GK = 1.0/( 1.0 + beta/beta_K );
    
    % Error calculation
    SpdErr = (GenSpd - RefGenSpd);

    % Integral calculation
    New_IntSpdErr = IntSpdErr + SpdErr*dt;

    % PID formula
    PitCon = (Kp * SpdErr + Ki * IntSpdErr) * GK;
    
    % Rate limiter
    PitConRate = (PitCon - beta) / dt;
    if PitConRate > MaxPitRat
        PitCon = beta + MaxPitRat * dt;
    elseif PitConRate < -MaxPitRat
        PitCon = beta - MaxPitRat * dt;
    end

    % Clamp the output
    if PitCon > MaxPit
        PitCon = MaxPit;
    elseif PitCon < MinPit
        PitCon = MinPit;
    else
        % Anti-windup
        IntSpdErr = New_IntSpdErr;
    end

    % Store state for the next iteration
    beta = PitCon;

    PitCon = reshape(PitCon, 1,1);
else
    if isempty(j)
        j = 1;
        PitCon = reshape(beta, 1,1);
        gainsOut = gainsIn;
        gainsOut(1) = Kp;
        gainsOut(2) = Ki;
    else
        PitCon = reshape(beta, 1,1);
        gainsOut = gainsIn;
        Kp = gainsOut(1);
        Ki = gainsOut(2);
    end
end


end

== matlab function SystemSimulationPPO/NREL PI Controller, 10Hz/MATLAB Function ==
  data: u input; y output
function y = fcn(u)
    for i=1:length(u)
        if u(i)>5
            u(i) = 5;
        else if u(i)<0.001
            u(i) = 0.001;
        else
            u(i) = u(i);
        end
    end
    y = u;
end

== matlab function SystemSimulationPPO/MATLAB Function ==
  data: x input; TowerDEL output; RotorDEL output; BladeDEL output
function [TowerDEL, RotorDEL, BladeDEL] = RainflowCountBaseline(x)
if isempty(x)
    TowerDEL = 0;
    RotorDEL = 0;
    BladeDEL = 0;
else
    TurbineLoads = x;
    rf_tower = rainflow(TurbineLoads(:,12)*1000,100);
    mT1 = 3;% S-N curve slope factor for steel
    mT2 = 5;
    towercycles = sum(rf_tower(:,1));
    N_ref = 5000000; % 
    stress_ref = 355e6*0.75;% 75% of Yield Strength for S355 steel
    Towerdamage_combined = 0;
    for i = 1:height(rf_tower)
        rangeT = rf_tower(i,2);
        countT = rf_tower(i,1);
        N_iT = N_ref*(stress_ref/rangeT)^mT2;
        if rangeT>stress_ref
            N_iT = N_ref*(stress_ref/rangeT)^mT1;
        end
    %N_iT = ((X_t+X_c-abs(2*lambda_ma*meanT-X_t+abs(X_c)))/(2*(lambda_mb)*rangeT))^m
        Towerdamage_combined = Towerdamage_combined + countT / N_iT;
    end
    %TowerLifeCycles = (1/Towerdamage_combined)*towercycles;
    TowerDEL = ( sum(rf_tower(:,1) .* rf_tower(:,2).^mT2) / towercycles )^(1/mT2);
% Rainflow count Rotor
    rf_rotor = rainflow(TurbineLoads(:,10)*1000,100);
    rotorcycles = sum(rf_rotor(:,1));
    mR1 = 3;% S-N curve slope factor for steel
    mR2 = 5;
    N_refR = 5000000; % Cycles to failure at stress of 90e6 Pa
    stress_refR = 355e6*0.75;% 75% of Yield Strength for S355 steel
    rotordamage_combined = 0;
    for i = 1:height(rf_rotor)
        rangeR = rf_rotor(i,2);
        countR = rf_rotor(i,1);
        N_iR = N_refR*(stress_refR/rangeR)^mR2;
        if rangeR > stress_refR
            N_iR = N_refR*(stress_refR/rangeR)^mR1;
        end
        rotordamage_combined = rotordamage_combined + countR / N_iR;
    end
    %rotorlifecycles = (1/rotordamage_combined)*rotorcycles;
    RotorDEL = ( sum(rf_rotor(:,1) .* rf_rotor(:,2).^mT2) / rotorcycles )^(1/mT2);
    % Rainflow edgewise and flapwise
    flapwiseMoment = TurbineLoads(:,14).*1000;
    edgewiseMoment = TurbineLoads(:,15).*1000;
    % Convert moments to stress time series (in Pa)
    % Optional: Total stress or worst-case
    bending_combined = sqrt(flapwiseMoment.^2 + edgewiseMoment.^2);
    % Now perform rainflow counting
    rf_combined = rainflow(bending_combined,100);
    % Define S-N curve parameters
    m = 9;             % typical for composites (higher than steel)
    X_t = 601.8e6;%793.05*10^6; % Tension strenght in Pa
    X_c = 407.3e6;%542.49*10^6; % Compression strength in Pa
    lambda_ma = 1.35*1.35*1.1*1.1*1; % partial safety factor short term strength
    lambda_mb = 1.35*1.1*1.2; % partial safety factor fatigue strength
    totalCycles=sum(rf_combined(:,1));
    damage_combined = 0;
    for i = 1:height(rf_combined)
        range = rf_combined(i,2);
        mean = rf_combined(i,3);
        count = rf_combined(i,1);
        N_i = ((X_t+X_c-abs(2*lambda_ma*mean-X_t+abs(X_c)))/(2*(lambda_mb)*range))^m;
        damage_combined = damage_combined + count / N_i;
    end
    %lifeCycles = (1/damage_combined)*totalCycles;
    BladeDEL = ( sum(rf_combined(:,1) .* rf_combined(:,2).^m) / totalCycles )^(1/m);
end
end

== matlab function SystemSimulationPPO/Cost Calculator/MATLAB Function ==
  data: DEL input; cost output; Pgen input; rotorspeed input
function cost  = fcn(DEL,Pgen,rotorspeed)
    if Pgen>4900
        powercost = 1;
    else
        powercost = Pgen*1000;
    end
    if rotorspeed>1.2671
        rotorspeedcost = 1.2671*1000000;
    else
        rotorspeedcost=1;
    end
    
    %rotorspeedcost = (-(rotorspeed-1.2671)^2)*200+1.2671;
    %if rotorspeedcost<0
        %rotorspeedcost=0;
    %else
        %rotorspeedcost=1.2671*1000000;
    %end
    TowerCost = abs(DEL(1));
    RotorCost = abs(DEL(2));
    BladeCost = abs(DEL(3));
    %stateCosts = [powerCost TowerCost RotorCost BladeCost];
    w = [1 0.01 0.5].*powercost;
    w = w.*rotorspeedcost;
    %costVec = stateCosts.*w;
    cost = -w(1)*TowerCost-w(2)*RotorCost-w(3)*BladeCost;
    
end

== matlab function SystemSimulationPPO/MATLAB Function1 ==
  data: u input; y output; windI input; windO output
function [y,windO] = fcn(u,windI)
persistent dtt oldWind;
if isempty(dtt)
    dtt=0.1;
    oldWind = 0;
end
if mod(u,dtt) == 0
    y = false;
    windO = windI;
    oldWind = windO;
else
    y = true;
    windO = oldWind;
end
end

== matlab function SystemSimulationPPO/NREL PI Controller, 10Hz/GenSpeed, rad//sec/MATLAB Function5 ==
  data: omega_r input; GenSpeed output
function GenSpeed = omega_g(omega_r)
    N = 97;
    GenSpeed = N * omega_r; 
end

== matlab function SystemSimulationPPO/MPC, 10Hz/PF/MATLAB Function2 ==
  data: Cp_Table input; Ct_Table input; Beta_Array input; TSR_Array input; beta_in input; omega_r_meas_in input; v_free_in input; Pg_in input; estimate output; Vx_in input
function estimate  = ParticleFilterfcn(Cp_Table, Ct_Table, Beta_Array, TSR_Array, beta_in, omega_r_meas_in, v_free_in, Pg_in, Vx_in)
%% Resampling Method 1: Faiyaz Ahmed Version:1, Assumption Multivariate NormPDF, and IID
%%
persistent n x_prior pi_prior estimate_dx pi_posterior x_hat

NumberOfStates = 3;
NumberOfParticles = 1000;
measurementSigma = 0.01;
sampleSigma = 0.01;

if isempty(n)
    n = 1;
    
    mu = [0; 0; 1.2671];
    Sigma = eye(NumberOfStates) * sampleSigma;
    z = randn(NumberOfStates, NumberOfParticles);
    x_prior = repmat(mu, 1, NumberOfParticles) + Sigma * z;
    
    pi_prior = ones(1, NumberOfParticles) .* 1/NumberOfParticles;
    pi_posterior = ones(1, NumberOfParticles);
    x_hat = ones(NumberOfStates, 1);
    estimate_dx = ones(NumberOfStates, NumberOfParticles);
end

% Measurement Update

dt = 0.01;

N = 97;
A = pi * 63^2;
rho = 1.2250;

% m_t = 350000 + 1.025538456000000e+05;
% k_t = 5.365709074998403e+05;
% c_t = 9.855500547940415e+03;

m_t = 350000+   1.2e+05;
k_t =5.5726e+05;
c_t = 1.0235e+04;

J_Drivetrain = 4.3787e+07;

v_Rave = v_free_in + 0;
omega_r_meas = omega_r_meas_in + 0;
beta = beta_in + 0;
Pg = Pg_in + 0;
Vx_meas = Vx_in + 0;

% Start
pi_posterior(1, :) = pi_prior(1, :) .* (normpdf(x_prior(2, :), Vx_meas, measurementSigma) .* normpdf(x_prior(3, :), omega_r_meas, measurementSigma));
pi_posterior(1,:) = pi_posterior(1,:)/sum(pi_posterior(1,:));

x_posterior = x_prior;
% End

% Time Update

% Start

%% Function f Start

for loop_mdl =1:NumberOfParticles
    x_d = x_posterior(1, loop_mdl);
    v_x = x_posterior(2, loop_mdl);
    omega_r = x_posterior(3, loop_mdl);
    
    v = v_Rave - 0;
    
    
    Tr = 0.5 * 1/omega_r * rho * A * v^3 * Coef(beta, omega_r, v, Cp_Table, Ct_Table, Beta_Array, TSR_Array, 1);
    Ft = 0.5 * rho * A * v^2 * Coef(beta, omega_r, v, Cp_Table, Ct_Table, Beta_Array, TSR_Array, 2);
    
    Tg = Pg/(N * omega_r);
    
    Tr = reshape(Tr, 1, 1);
    Ft = reshape(Ft, 1, 1);
    Tg = reshape(Tg, 1, 1);
    
    estimate_dx(1, loop_mdl) = v_x;
    estimate_dx(2, loop_mdl) = (1/m_t) * ( Ft - c_t*v_x - k_t*x_d );
    estimate_dx(3, loop_mdl) = (1/(J_Drivetrain)) * ( Tr - N*Tg );
    
    x_prior(:, loop_mdl) = x_posterior(:, loop_mdl) + estimate_dx(:, loop_mdl)*dt;
end

% Function f End


%% Function End
pi_prior(1, :) = 1/NumberOfParticles;

% End

x_hat(:,1) = x_prior(:, :) * pi_posterior(1,:)';

% Resample
mu = [x_hat(1); x_hat(2); x_hat(3)];
Sigma = eye(NumberOfStates) * sampleSigma;
z = randn(NumberOfStates, NumberOfParticles);
x_prior = repmat(mu, 1, NumberOfParticles) + Sigma * z;

estimate = reshape(x_hat, 3, 1);
end


function [C]   = Coef(beta, omega_r, v, Cp_Table, Ct_Table, Beta_Array, TSR_Array, type)

R = 63;
tsr =  ((omega_r * R)/v);
tsr = round(tsr*10)/10;
beta = round(beta*10)/10;

tsr = max(tsr, 0);
tsr = min(tsr, 20);

beta = max(beta, 0);
beta = min(beta, 45);

if type == 1
    C_p = Cp_Table(TSR_Array == tsr, Beta_Array == beta);
    C = C_p;
else
    C_t = Ct_Table(TSR_Array == tsr, Beta_Array == beta);
    C = C_t;
end

end

== matlab function SystemSimulationPPO/MPC, 10Hz/UKF/MATLAB Function2 ==
  data: Cp_Table input; estimate output; Ct_Table input; Beta_Array input; TSR_Array input; beta_in input; omega_r_meas_in input; v_free_in input; Pg_in input; Vx_in input
function estimate = UKF( Cp_Table, Ct_Table, Beta_Array, TSR_Array, beta_in, omega_r_meas_in, v_free_in, Pg_in,  Vx_in)

persistent n numberOfStates numberofSigmaPoints numberofMeasurements
persistent x_posterior x_prior sigma_x_prior sigma_x_posterior
persistent sigma_y_prior y_hat_prior estimate_dx x_hat
persistent P_x_posterior P_x_prior P_y_prior P_xy_prior
persistent K_gain Wm Wc Rv Rn eta


if isempty(n)
    
    n=1;
    
    % Initialize Sigma Points
    numberOfStates = 3;
    numberofSigmaPoints = 2*numberOfStates + 1;
    numberofMeasurements = 2;
    
    initialValues = [0; 0; 1.2671];
    
    x_posterior = zeros(numberOfStates, 1) + initialValues;             % Initial estimate of state variables
    x_prior = zeros(numberOfStates, 1);
    
    
    sigma_x_prior = zeros(numberOfStates, numberofSigmaPoints);
    sigma_x_posterior = zeros(numberOfStates, numberofSigmaPoints);
    
    sigma_y_prior = zeros(numberofMeasurements, numberofSigmaPoints);
    y_hat_prior = zeros(numberofMeasurements, 1);
    
    alpha = 1e-3;                                                       % Determines the spread of the sigma points, le-4 < alpha < 1
    K_gain = eye(numberOfStates, numberofMeasurements);
    
    P_x_posterior = eye(numberOfStates)*alpha;                          % Initial state covariance matrix, (alpha because it's a small number, haha)
    P_x_prior = eye(numberOfStates);                                    % Initial state covariance matrix
    P_y_prior = eye(numberofMeasurements);
    P_xy_prior = ones(numberOfStates,numberofMeasurements);
    
    beta = 2;                                                           % beta = 2, optimal for Gaussian
    %         kappa = 0;                                                        % kappa = 0 or 3-L (Kappa is used in a different way of calculating the weights)
    lambda = numberOfStates * (alpha^2 - 1);                            % or lambda = alpha^2 * (L + kappa) - L, composite scaling parameter
    c = numberOfStates + lambda;
    eta = sqrt(numberOfStates + lambda);                                % Yet another scaling parameter
    
    Wm = zeros(1,numberofSigmaPoints);                                  % Weights for sigma points
    Wc = zeros(1,numberofSigmaPoints);                                  % Weights for covariance matricies
    Wm(1, 1) = lambda/c;
    Wc(1, 1) = lambda/c + (1-alpha^2+beta);
    
    for i = 2:2*numberOfStates+1
        Wm(1, i) = 1/(2*c);
        Wc(1, i) = 1/(2*c);
    end
    
    estimate_dx = zeros(numberOfStates, numberofSigmaPoints);
    
    processCovariance= 0.01;
    measurementCovariance = 0.01;
    
    Rv = eye(numberOfStates) * processCovariance;                  % Process covariance matrix, guess
    Rn = eye(numberofMeasurements) * measurementCovariance;        % Measurement noise covariance matrix, guess
end

%%
% Time Update Start

% Sigma Posterior Definition Start
sigma_x_posterior(:, 1) = x_posterior(:, 1);
temp_sqrt = eta * chol(P_x_posterior);
temp_repmat = repmat(x_posterior(:, 1), 1, numberOfStates);
sigma_x_posterior(:, 2:numberOfStates+1) = temp_repmat + temp_sqrt;
sigma_x_posterior(:, numberOfStates+2:2*numberOfStates+1) = temp_repmat - temp_sqrt;
% Sigma Posterior Definition End

%% Function f Start

dt = 0.01;

N = 97;
A = pi * 63^2;
rho = 1.2250;

%     m_t = 350000 + 1.025538456000000e+05;
%     k_t = 5.365709074998403e+05;
%     c_t = 9.855500547940415e+03;

m_t =  (350000+   1.2e+05);
k_t =  (5.5726e+05);
c_t =  (1.0235e+04);

J_Drivetrain = 4.3787e+07;

v_Rave = v_free_in + 0;
omega_r_meas = omega_r_meas_in + 0;
beta = beta_in + 0;
Pg = Pg_in + 0;
Vx_meas = Vx_in + 0;

for loop_mdl =1:numberofSigmaPoints
    
    x_d = sigma_x_posterior(1, loop_mdl);
    v_x = sigma_x_posterior(2, loop_mdl);
    omega_r = sigma_x_posterior(3, loop_mdl);
    
    v = v_Rave - 0;
    
    Tr = 0.5 * 1/omega_r * rho * A * v^3 * Coef(beta, omega_r, v, Cp_Table, Ct_Table, Beta_Array, TSR_Array, 1);
    Ft = 0.5 * rho * A * v^2 * Coef(beta, omega_r, v, Cp_Table, Ct_Table, Beta_Array, TSR_Array, 2);
    
    Tr = reshape(Tr, 1, 1);
    Ft = reshape(Ft, 1, 1);
    
    Tg = Pg/(N * omega_r);
    Tg = reshape(Tg, 1, 1);
    
    estimate_dx(1, loop_mdl) = v_x;
    estimate_dx(2, loop_mdl) = (1/m_t) * ( Ft - c_t*v_x - k_t*x_d );
    estimate_dx(3, loop_mdl) = (1/J_Drivetrain) * ( Tr - N*Tg ) ;
    
    sigma_x_prior(:, loop_mdl) = sigma_x_posterior(:, loop_mdl) + estimate_dx(:, loop_mdl)*dt;               % + sum(normrnd(0, Rv), 2);
end

% Function f End
%%
x_prior = ( Wm * sigma_x_prior')';

P_x_prior = P_x_prior * 0;
for loop_Px=1:numberofSigmaPoints
    P_x_prior = P_x_prior + Wc(1, loop_Px) * (sigma_x_prior(:, loop_Px) - x_prior) * (sigma_x_prior(:, loop_Px) - x_prior)';
end
P_x_prior = P_x_prior + Rv;

sigma_y_prior = sigma_x_prior(2:3, :);                              %+ normrnd(0, Rn); measurement estimate

y_hat_prior = (Wm * sigma_y_prior')';

% Time Update End

%% Measurement Update Start

P_y_prior = P_y_prior * 0;
for loop_Py=1:numberofSigmaPoints
    P_y_prior = P_y_prior + Wc(1, loop_Py) * (sigma_y_prior(:, loop_Py) - y_hat_prior) * (sigma_y_prior(:, loop_Py) - y_hat_prior)';
end
P_y_prior = P_y_prior + Rn;


P_xy_prior = P_xy_prior * 0;
for loop_Pxy=1:numberofSigmaPoints
    P_xy_prior = P_xy_prior + Wc(1, loop_Pxy) * (sigma_x_prior(:, loop_Pxy) - x_prior) * (sigma_y_prior(:, loop_Pxy) - y_hat_prior)';
end

K_gain = P_xy_prior / P_y_prior;

x_posterior(:, 1) = x_prior + K_gain * ([Vx_meas; omega_r_meas] - y_hat_prior);

P_x_posterior = P_x_prior - K_gain * P_y_prior * K_gain';

x_hat = x_posterior;

% Measurement Udate End

estimate = reshape(x_hat, 3, 1);
end



function [C]   = Coef(beta, omega_r, v, Cp_Table, Ct_Table, Beta_Array, TSR_Array, type)

R = 63;
tsr =  ((omega_r * R)/v);
tsr = round(tsr*10)/10;
beta = round(beta*10)/10;

tsr = max(tsr, 0);
tsr = min(tsr, 20);

beta = max(beta, 0);
beta = min(beta, 45);

if type == 1
    C_p = Cp_Table(TSR_Array == tsr, Beta_Array == beta);
    C = C_p;
else
    C_t = Ct_Table(TSR_Array == tsr, Beta_Array == beta);
    C = C_t;
end

end
